simulink model "p2_simulink"  (R2020b)
settings: Solver=VariableStepAuto  StartTime=0.0  StopTime=15  MaxStep=0.001  RelTol=1e-4
values from neighbouring files (symbols this model uses):
  L = 0.6    [p2.m]
libraries: simulink x1
settings Model: Creator=35193  LastModifiedBy=35193
settings SolverCC: ZeroCrossAlgorithm=Adaptive
settings DebuggingCC: IgnoredZcDiagnostic=none

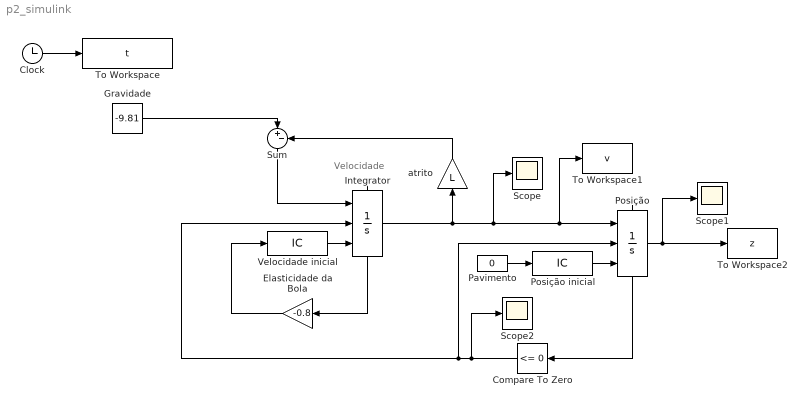
== system p2_simulink ==
  note: Velocidade
  Clock : Clock
  Compare To Zero : simulink/Logic and Bit Operations/Compare To Zero  relop=<=  OutDataTypeStr=boolean
  Elasticidade da Bola : Gain  Gain=-0.8
  Gravidade : Constant  Value=-9.81
  Integrator : Integrator  ExternalReset=rising  InitialConditionSource=external  ShowStatePort=on
  Pavimento : Constant  Value=0
  Posição : Integrator  ExternalReset=rising  InitialConditionSource=external  ShowStatePort=on
  Posição inicial : InitialCondition  Value=10
  Scope : Scope
  Scope1 : Scope
  Scope2 : Scope
  Sum : Sum  Inputs=|+-
  To Workspace : ToWorkspace  VariableName=t  SampleTime=-1
      settings: Save2DSignal=2-D array (concatenate along first dimension)
  To Workspace1 : ToWorkspace  VariableName=v  SampleTime=-1
      settings: Save2DSignal=2-D array (concatenate along first dimension)
  To Workspace2 : ToWorkspace  VariableName=z  SampleTime=-1
      settings: Save2DSignal=2-D array (concatenate along first dimension)
  Velocidade inicial : InitialCondition  Value=0
  atrito : Gain  Gain=L
  wires:
  Clock/1 -> To Workspace/1
  Integrator/State -> Elasticidade da Bola/1
  Posição/State -> Compare To Zero/1
  Compare To Zero/1 -> Scope2/1, Posição/2, Integrator/2
  Posição inicial/1 -> Posição/3
  Pavimento/1 -> Posição inicial/1
  Velocidade inicial/1 -> Integrator/3
  Elasticidade da Bola/1 -> Velocidade inicial/1
  Posição/1 -> Scope1/1, To Workspace2/1
  Integrator/1 -> atrito/1, Scope/1, To Workspace1/1, Posição/1
  atrito/1 -> Sum/2
  Gravidade/1 -> Sum/1
  Sum/1 -> Integrator/1
